simulink model "open_loop"  (R2017a)
settings: Solver=FixedStepAuto  StartTime=0.0  StopTime=500  FixedStep=0.01  RelTol=1e-3
libraries: simulink x1
settings Model: Creator=Sidharth Agarwal  LastModifiedBy=Sidharth Agarwal

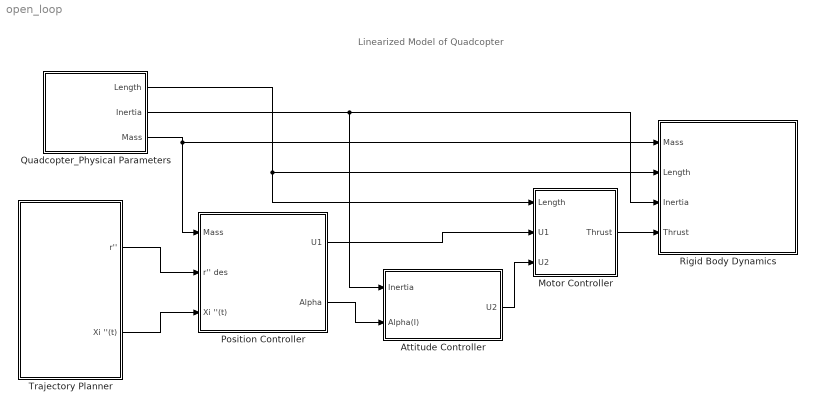
== system open_loop ==
  note: Linearized Model of Quadcopter
  Attitude Controller : Subsystem
  Motor Controller : Subsystem
  Position Controller : Subsystem
  Quadcopter_Physical Parameters : Subsystem
  Rigid Body Dynamics : Subsystem
  Trajectory Planner : Subsystem
  wires:
  Trajectory Planner/2(Xi ''(t)) -> Position Controller/3(Xi ''(t))
  Motor Controller/1(Thrust) -> Rigid Body Dynamics/4(Thrust)
  Trajectory Planner/1(r'') -> Position Controller/2(r'' des)
  Attitude Controller/1(" U2 ") -> Motor Controller/3(U2)
  Quadcopter_Physical Parameters/2(Inertia) -> Rigid Body Dynamics/3(Inertia), Attitude Controller/1(Inertia)
  Quadcopter_Physical Parameters/3(Mass) -> Rigid Body Dynamics/1(Mass), Position Controller/1(Mass)
  Position Controller/1(U1) -> Motor Controller/2(U1)
  Position Controller/2(Alpha) -> Attitude Controller/2(Alpha(I))
  Quadcopter_Physical Parameters/1(Length) -> Motor Controller/1(Length), Rigid Body Dynamics/2("Length ")

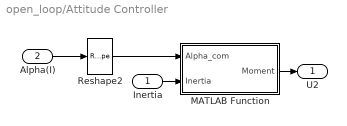
== system open_loop/Attitude Controller ==
  Inertia : Inport
  Alpha(I) : Inport  Port=2
  MATLAB Function : MATLAB Function  TreatAsAtomicUnit=on
  Reshape2 : Reshape  OutputDimensionality=Column vector (2-D)
  " U2 " : Outport
  wires:
  Alpha(I)/1 -> Reshape2/1
  Reshape2/1 -> MATLAB Function/1(Alpha_com)
  MATLAB Function/1(Moment) -> " U2 "/1
  Inertia/1 -> MATLAB Function/2(Inertia)

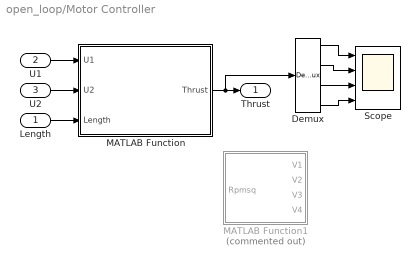
== system open_loop/Motor Controller ==
  Length : Inport
  U1 : Inport  Port=2
  U2 : Inport  Port=3
  Demux : Demux
  MATLAB Function : MATLAB Function  TreatAsAtomicUnit=on
  MATLAB Function1 : MATLAB Function  Commented=on  TreatAsAtomicUnit=on
  Scope : Scope  NumInputPorts=4
  Thrust : Outport
  wires:
  U2/1 -> MATLAB Function/2(U2)
  Length/1 -> MATLAB Function/3(Length)
  U1/1 -> MATLAB Function/1(U1)
  MATLAB Function/1(Thrust) -> Demux/1, Thrust/1
  Demux/4 -> Scope/4
  Demux/1 -> Scope/1
  Demux/2 -> Scope/2
  Demux/3 -> Scope/3

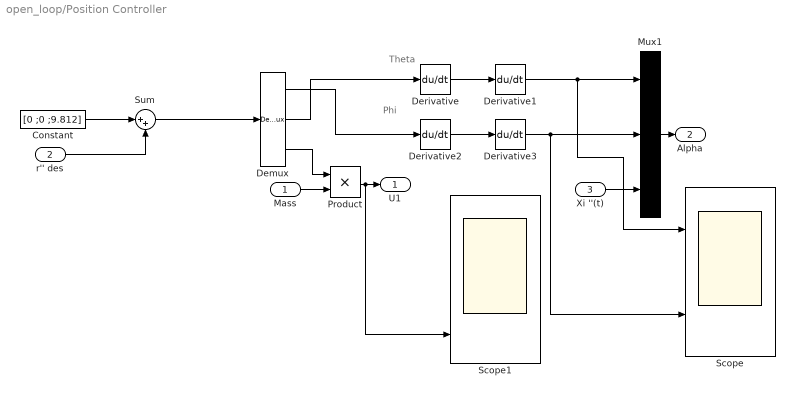
== system open_loop/Position Controller ==
  note: Phi
  note: Theta
  Mass : Inport
  r'' des : Inport  Port=2
  Xi ''(t) : Inport  Port=3
  Constant : Constant  Value=[0 ;0 ;9.812]
  Demux : Demux  Outputs=3
  Derivative{,1..3} (4 alike) : Derivative
  Mux1 : Mux  Inputs=3
  Product : Product
  Scope : Scope  NumInputPorts=2
  Scope1 : Scope  NumInputPorts=3
  Sum : Sum  Inputs=|++
  U1 : Outport
  Alpha : Outport  Port=2
  wires:
  Xi ''(t)/1 -> Mux1/3
  Mux1/1 -> Alpha/1
  Mass/1 -> Product/2
  Demux/3 -> Product/1
  Product/1 -> Scope1/3, U1/1
  Sum/1 -> Demux/1
  Constant/1 -> Sum/1
  r'' des/1 -> Sum/2
  Derivative/1 -> Derivative1/1
  Derivative1/1 -> Scope/1, Mux1/1
  Derivative2/1 -> Derivative3/1
  Derivative3/1 -> Scope/2, Mux1/2
  Demux/1 -> Derivative2/1
  Demux/2 -> Derivative/1

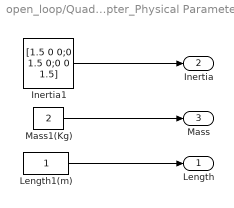
== system open_loop/Quadcopter_Physical Parameters ==
  Inertia1 : Constant  Value=[1.5 0 0;0 1.5 0;0 0 1.5]
  Length1(m) : Constant
  Mass1(Kg) : Constant  Value=2
  Length : Outport
  Inertia : Outport  Port=2
  Mass : Outport  Port=3
  wires:
  Inertia1/1 -> Inertia/1
  Mass1(Kg)/1 -> Mass/1
  Length1(m)/1 -> Length/1

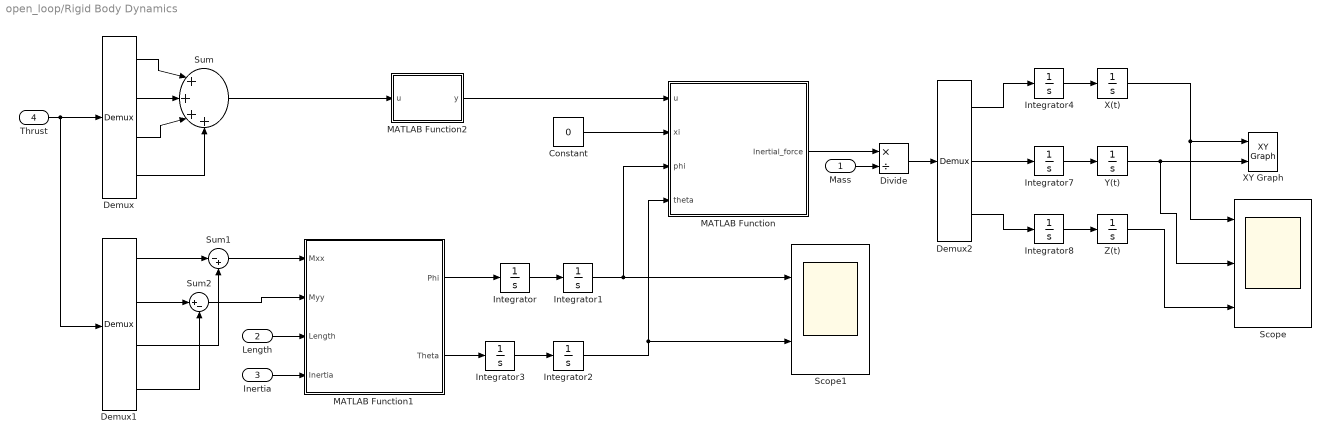
== system open_loop/Rigid Body Dynamics ==
  Mass : Inport
  "Length " : Inport  Port=2
  Inertia : Inport  Port=3
  Thrust : Inport  Port=4
  Constant : Constant  Value=0
  Demux : Demux
  Demux1 : Demux
  Demux2 : Demux  Outputs=3
  Divide : Product  Inputs=*/
  Integrator{,1..4,7..8} (7 alike) : Integrator
  MATLAB Function : MATLAB Function  TreatAsAtomicUnit=on
  MATLAB Function1 : MATLAB Function  TreatAsAtomicUnit=on
  MATLAB Function2 : MATLAB Function  TreatAsAtomicUnit=on
  Scope : Scope  NumInputPorts=3
  Scope1 : Scope  NumInputPorts=2
  Sum : Sum  Inputs=|++++
  Sum1 : Sum  Inputs=|-+
  Sum2 : Sum  Inputs=|+-
  X(t) : Integrator
  XY Graph : simulink/Sinks/XY Graph  xmin=-20  xmax=900  ymin=-20  ymax=50  st=-1
  Y(t) : Integrator
  Z(t) : Integrator
  wires:
  Thrust/1 -> Demux1/1, Demux/1
  Demux/1 -> Sum/1
  Demux/2 -> Sum/2
  Demux/3 -> Sum/3
  Demux/4 -> Sum/4
  Sum/1 -> MATLAB Function2/1(u)
  MATLAB Function2/1(y) -> MATLAB Function/1(u)
  Demux1/1 -> Sum1/1
  Demux1/3 -> Sum1/2
  Demux1/2 -> Sum2/1
  Demux1/4 -> Sum2/2
  Constant/1 -> MATLAB Function/2(xi)
  "Length "/1 -> MATLAB Function1/3(Length)
  Inertia/1 -> MATLAB Function1/4(Inertia)
  MATLAB Function1/1(Phi) -> Integrator/1
  Integrator3/1 -> Integrator2/1
  Integrator/1 -> Integrator1/1
  MATLAB Function1/2(Theta) -> Integrator3/1
  Integrator1/1 -> MATLAB Function/3(phi), Scope1/1
  MATLAB Function/1(Inertial_force) -> Divide/1
  Mass/1 -> Divide/2
  Divide/1 -> Demux2/1
  Demux2/1 -> Integrator4/1
  Integrator4/1 -> X(t)/1
  Demux2/2 -> Integrator7/1
  Integrator7/1 -> Y(t)/1
  Integrator8/1 -> Z(t)/1
  Demux2/3 -> Integrator8/1
  X(t)/1 -> Scope/1, XY Graph/1
  Y(t)/1 -> Scope/2, XY Graph/2
  Z(t)/1 -> Scope/3
  Integrator2/1 -> MATLAB Function/4(theta), Scope1/2
  Sum1/1 -> MATLAB Function1/1(Mxx)
  Sum2/1 -> MATLAB Function1/2(Myy)

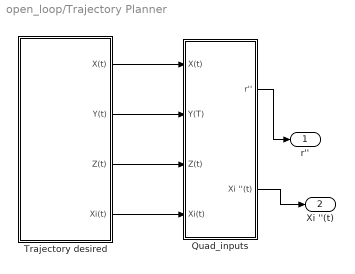
== system open_loop/Trajectory Planner ==
  Quad_inputs : Subsystem
  Trajectory desired : Subsystem
  r'' : Outport
  Xi ''(t) : Outport  Port=2
  wires:
  Quad_inputs/1(r'') -> r''/1
  Quad_inputs/2(Xi ''(t)) -> Xi ''(t)/1
  Trajectory desired/1(X(t)) -> Quad_inputs/1(X(t))
  Trajectory desired/2(Y(t)) -> Quad_inputs/2(Y(T))
  Trajectory desired/3(Z(t)) -> Quad_inputs/3(Z(t))
  Trajectory desired/4(Xi(t)) -> Quad_inputs/4(Xi(t))

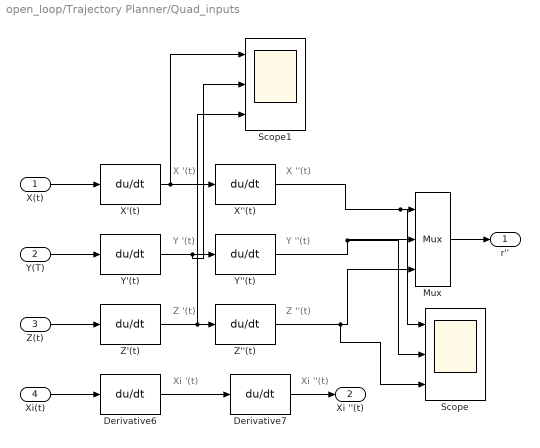
== system open_loop/Trajectory Planner/Quad_inputs ==
  note: Xi ''(t)
  note: X '(t)
  note: Y '(t)
  note: Z '(t)
  note: Xi '(t)
  note: X ''(t)
  note: Y ''(t)
  note: Z ''(t)
  X(t) : Inport
  Y(T) : Inport  Port=2
  Z(t) : Inport  Port=3
  Xi(t) : Inport  Port=4
  Derivative6 : Derivative
  Derivative7 : Derivative
  Mux : Mux  Inputs=3
  Scope : Scope  NumInputPorts=3
  Scope1 : Scope  NumInputPorts=3
  X''(t) : Derivative
  X'(t) : Derivative  CoefficientInTFapproximation=1
  Y''(t) : Derivative  CoefficientInTFapproximation=1
  Y'(t) : Derivative  CoefficientInTFapproximation=1
  Z''(t) : Derivative
  Z'(t) : Derivative
  r'' : Outport
  Xi ''(t) : Outport  Port=2
  wires:
  X(t)/1 -> X'(t)/1
  X'(t)/1 -> X''(t)/1, Scope1/1
  Y'(t)/1 -> Scope1/2, Y''(t)/1
  Y(T)/1 -> Y'(t)/1
  Z'(t)/1 -> Scope1/3, Z''(t)/1
  Z(t)/1 -> Z'(t)/1
  Derivative6/1 -> Derivative7/1
  Xi(t)/1 -> Derivative6/1
  X''(t)/1 -> Scope/1, Mux/1
  Y''(t)/1 -> Scope/2, Mux/2
  Z''(t)/1 -> Scope/3, Mux/3
  Mux/1 -> r''/1
  Derivative7/1 -> Xi ''(t)/1

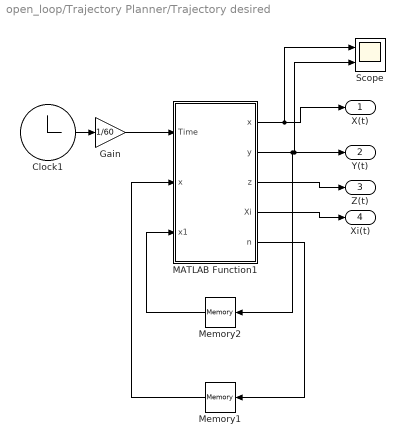
== system open_loop/Trajectory Planner/Trajectory desired ==
  Clock1 : Clock
  Gain : Gain  Gain=1/60
  MATLAB Function1 : MATLAB Function  TreatAsAtomicUnit=on
  Memory1 : Memory
  Memory2 : Memory
  Scope : Scope  NumInputPorts=2
  X(t) : Outport
  Y(t) : Outport  Port=2
  Z(t) : Outport  Port=3
  Xi(t) : Outport  Port=4
  wires:
  MATLAB Function1/4(Xi) -> Xi(t)/1
  MATLAB Function1/1(x) -> Scope/1, X(t)/1
  Clock1/1 -> Gain/1
  Memory1/1 -> MATLAB Function1/2("x ")
  Gain/1 -> MATLAB Function1/1(Time)
  MATLAB Function1/5(n) -> Memory1/1
  Memory2/1 -> MATLAB Function1/3(x1)
  MATLAB Function1/2(y) -> Memory2/1, Scope/2, Y(t)/1
  MATLAB Function1/3(z) -> Z(t)/1

== matlab function open_loop/Motor Controller/MATLAB Function ==
  data: U1 input; U2 input; Thrust output; Length input
function Thrust = fcn(U1, U2, Length)

B=[U1;U2(1)/(Length);U2(2)/(Length);U2(3)];
Ainv=[0.25 0.5 0 0.25;0.25 0 0.5 -0.25;0.25 -0.5 0  0.25;0.25 0 -0.5 -0.25];
Thrust=Ainv*B;
end

== matlab function open_loop/Attitude Controller/MATLAB Function ==
  data: Alpha_com input; Moment output; Inertia input
function Moment = fcn(Alpha_com,Inertia)

 Moment=[Alpha_com(1)*Inertia(1,1);Alpha_com(2)*Inertia(2,2);Alpha_com(3)*Inertia(3,3)];

== matlab function open_loop/Motor Controller/MATLAB Function1 ==
  data: Rpmsq input; V1 output; V2 output; V3 output; V4 output
function [V1,V2,V3,V4] = fcn(Rpmsq)
%   Here rpmsq versus voltage relation is used

== matlab function open_loop/Rigid Body Dynamics/MATLAB Function ==
  data: u input; xi input; Inertial_force output; phi input; theta input
function Inertial_force = Rotation(u,xi,phi,theta)

Rx=[1,0,0;0,cos(phi),-sin(phi);0,sin(phi),cos(phi)];
Ry=[cos(theta),0,sin(theta);0,1,0;-sin(theta),0,cos(theta)];
Rz=[cos(xi),-sin(xi),0;sin(xi),cos(xi),0;0,0,1];
Rib=(Rx*Ry*Rz);
Inertial_force = Rib*u;
end

== matlab function open_loop/Rigid Body Dynamics/MATLAB Function1 ==
  data: Mxx input; Phi output; Myy input; Length input; Inertia input; Theta output
function [Phi,Theta] = Alpha(Mxx,Myy,Length,Inertia)

Phi= (Mxx*Length)/Inertia(1,1);
Theta=(Myy*Length)/Inertia(2,2);
end

== matlab function open_loop/Rigid Body Dynamics/MATLAB Function2 ==
  data: u input; y output
function y = fcn(u)

y = [0;0;u];

== matlab function open_loop/Trajectory Planner/Trajectory desired/MATLAB Function1 ==
  data: x output; y output; z output; Xi output; n output; Time input; x input; x1 input

function [x,y,z,Xi,n] =fcn(Time,x,x1)
period=6;
z=0;
Xi=0;
n=x;

   if Time==(n+1)*period
       n=n+1;
       
    end
time=Time-n*period; 
    if time<=1.5
        x=7.90123456790123*time^5-29.6296296296296*time^4+29.6296296296296*time^3;
        y=x1;
        
    elseif time<=3
        x=10;
        y=3.95061728395062*time^5-44.4444444444*time^4+192.592592592593*time^3-400*time^2+400*time-155+10*n;
        
      
    elseif time<=4.5
        x=-7.90123456790123*time^5+148.148148148148*time^4-1096.29629629630*time^3+4000*time^2-7200*time+5130;
        y=x1;
    else 
       x=0;
       y=3.95061728395062*time^5-103.703703703704*time^4+1081.48148148148*time^3-5600*time^2+14400*time-14710+10*n;
       
       
    end
  
end
